simulink model "OFDM_Transreceiver"  (R2020b)
settings: Solver=VariableStepAuto  StartTime=0.0  StopTime=5000  RelTol=1e-3
libraries: xbsIndex_r4 x21, commchan3 x1, commrandsrc3 x1, commsink2 x1
settings Model: Creator=Gokaraan  LastModifiedBy=Gokaraan

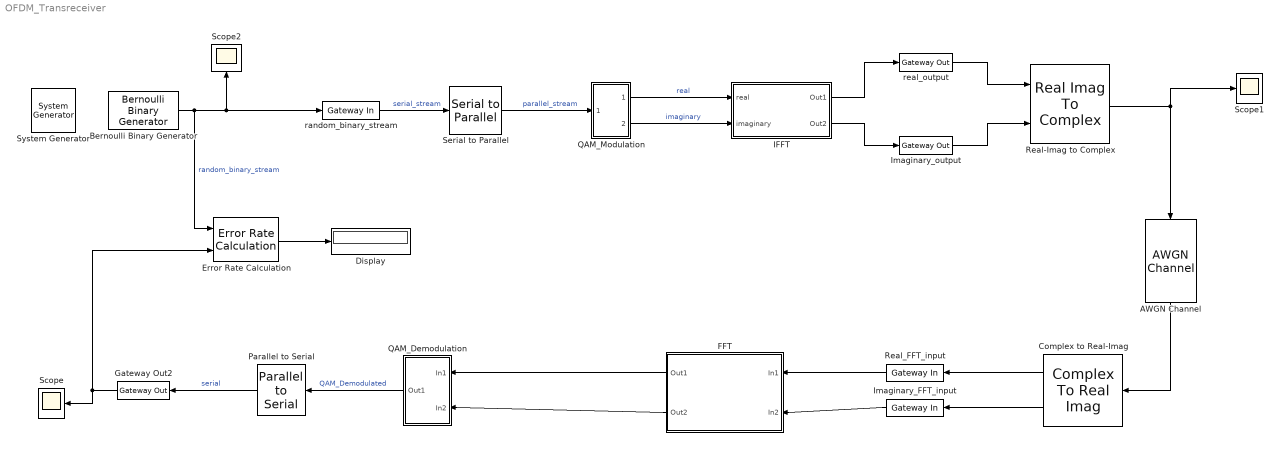
== system OFDM_Transreceiver ==
  " System Generator" : xbsIndex_r4/ System Generator  Tag=genX  xilinxfamily=artix7  part=xc7a35ti  speed=-1L  package=cpg236  synthesis_tool=Vivado  clock_wrapper=Clock Enables  directory=C:/Users/Gokaraan/Documents/Composer/OFDM/HDL  proj_type=Vivado  Synth_file=Vivado Synthesis Defaults  Impl_file=Vivado Implementation Defaults  testbench=off  simulink_period=1  sysclk_period=10  dcm_input_clock_period=10  incr_netlist=off  trim_vbits=Everywhere in SubSystem  dbl_ovrd=According to Block Masks  core_generation=According to Block Masks  run_coregen=off  deprecated_control=off  eval_field=0  block_type=sysgen
  AWGN Channel : commchan3/AWGN Channel  InputProcessing=Columns as channels (frame based)  seed=67  noiseMode="Signal to noise ratio  (SNR)"  EbNodB=10  EsNodB=10  SNRdB=70  bitsPerSym=1  Ps=1  Tsym=1  variance=1
  Bernoulli Binary Generator : commrandsrc3/Bernoulli Binary Generator  ProbabilityOfZero=0.5  SeedSource=Parameter  Seed=61  SampleTime=1  SamplesPerFrame=1  OutputDataType=double  SimulateUsing=Interpreted execution
  Complex to Real-Imag : ComplexToRealImag
  Display : Display
  Error Rate Calculation : commsink2/Error Rate Calculation  N=1672  st_delay=700  cp_mode=Entire frame  subframe=[]  PMode=Port  WsName=ErrorVec  RsMode2=off  stop=off  numErr=100  maxBits=1e6
      settings: SourceProductName=Communications Toolbox
  FFT : Subsystem
  Gateway Out2 : xbsIndex_r4/Gateway Out  inherit_from_input=off  hdl_port=on  rows=1  columns=1  UseAsDAC=off  DACChannel='1'  interface=None  automatic_assignment=on  address_offset=hex2dec('00')  intf_name=''  intf_description=''  timing_constraint=None  locs_specified=off  LOCs={}  io_standard={}  block_type=gatewayout
  IFFT : Subsystem
  Imaginary_FFT_input : xbsIndex_r4/Gateway In  gui_display_data_type=Fixed-point  arith_type="Signed  (2's comp)"  n_bits=16  bin_pt=15  preci_type=Single  exp_width=8  frac_width=24  rows=1  columns=1  quantization="Round  (unbiased: +/- Inf)"  overflow=Saturate  period=4  UseAsADC=off  ADCChannel='1'  interface=None  automatic_assignment=on  address_offset=hex2dec('00')  intf_name=''  intf_description=''  default_value=0  timing_constraint=None  locs_specified=off  LOCs={}  io_standard={}  inherit_from_input=off  hdl_port=on  dbl_ovrd=off  block_type=gatewayin
  Imaginary_output : xbsIndex_r4/Gateway Out  inherit_from_input=off  hdl_port=on  rows=1  columns=1  UseAsDAC=off  DACChannel='1'  interface=None  automatic_assignment=on  address_offset=hex2dec('00')  intf_name=''  intf_description=''  timing_constraint=None  locs_specified=off  LOCs={}  io_standard={}  block_type=gatewayout
  Parallel to Serial : xbsIndex_r4/Parallel to Serial  output_order=Least Significant Word First  arith_type=Unsigned  output_bits=1  bin_pt=0  rst=off  en=off  latency=1  dbl_ovrd=off  block_type=p2s
      settings: infoedit=Each sample presented at the input becomes several samples presented serially at the output.
  QAM_Demodulation : Subsystem
  QAM_Modulation : Subsystem
  Real-Imag to Complex : RealImagToComplex
  Real_FFT_input : xbsIndex_r4/Gateway In  gui_display_data_type=Fixed-point  arith_type="Signed  (2's comp)"  n_bits=16  bin_pt=15  preci_type=Single  exp_width=8  frac_width=24  rows=1  columns=1  quantization="Round  (unbiased: +/- Inf)"  overflow=Saturate  period=4  UseAsADC=off  ADCChannel='1'  interface=None  automatic_assignment=on  address_offset=hex2dec('00')  intf_name=''  intf_description=''  default_value=0  timing_constraint=None  locs_specified=off  LOCs={}  io_standard={}  inherit_from_input=off  hdl_port=on  dbl_ovrd=off  block_type=gatewayin
  Scope : Scope
  Scope1 : Scope
  Scope2 : Scope
  Serial to Parallel : xbsIndex_r4/Serial to Parallel  input_order=Least Significant Word First  arith_type=Unsigned  output_bits=4  bin_pt=0  rst=off  en=off  latency=1  dbl_ovrd=off  block_type=s2p
      settings: infoedit=Groups of samples presented serially at the input become single samples presented at the output.
  random_binary_stream : xbsIndex_r4/Gateway In  gui_display_data_type=Fixed-point  arith_type=Unsigned  n_bits=1  bin_pt=0  preci_type=Single  exp_width=8  frac_width=24  rows=1  columns=1  quantization="Round  (unbiased: +/- Inf)"  overflow=Saturate  period=1  UseAsADC=off  ADCChannel='1'  interface=None  automatic_assignment=on  address_offset=hex2dec('00')  intf_name=''  intf_description=''  default_value=0  timing_constraint=None  locs_specified=off  LOCs={}  io_standard={}  inherit_from_input=off  hdl_port=on  dbl_ovrd=off  block_type=gatewayin
  real_output : xbsIndex_r4/Gateway Out  inherit_from_input=off  hdl_port=on  rows=1  columns=1  UseAsDAC=off  DACChannel='1'  interface=None  automatic_assignment=on  address_offset=hex2dec('00')  intf_name=''  intf_description=''  timing_constraint=None  locs_specified=off  LOCs={}  io_standard={}  block_type=gatewayout
  wires:
  Bernoulli Binary Generator/1 -> Error Rate Calculation/1, random_binary_stream/1, Scope2/1  "random_binary_stream"
  Complex to Real-Imag/2 -> Imaginary_FFT_input/1
  random_binary_stream/1 -> Serial to Parallel/1  "serial_stream"
  Complex to Real-Imag/1 -> Real_FFT_input/1
  Imaginary_output/1 -> Real-Imag to Complex/2
  AWGN Channel/1 -> Complex to Real-Imag/1
  Real-Imag to Complex/1 -> Scope1/1, AWGN Channel/1
  Parallel to Serial/1 -> Gateway Out2/1  "serial"
  Gateway Out2/1 -> Scope/1, Error Rate Calculation/2
  real_output/1 -> Real-Imag to Complex/1
  Error Rate Calculation/1 -> Display/1
  Serial to Parallel/1 -> QAM_Modulation/1(In1)  "parallel_stream"
  QAM_Modulation/1(Out1) -> IFFT/1(real)  "real"
  QAM_Modulation/2(Out2) -> IFFT/2(imaginary)  "imaginary"
  IFFT/1(Out1) -> real_output/1
  IFFT/2(Out2) -> Imaginary_output/1
  Real_FFT_input/1 -> FFT/1(In1)
  Imaginary_FFT_input/1 -> FFT/2(In2)
  FFT/1(Out1) -> QAM_Demodulation/1(In1)
  FFT/2(Out2) -> QAM_Demodulation/2(In2)
  QAM_Demodulation/1(Out1) -> Parallel to Serial/1  "QAM_Demodulated"

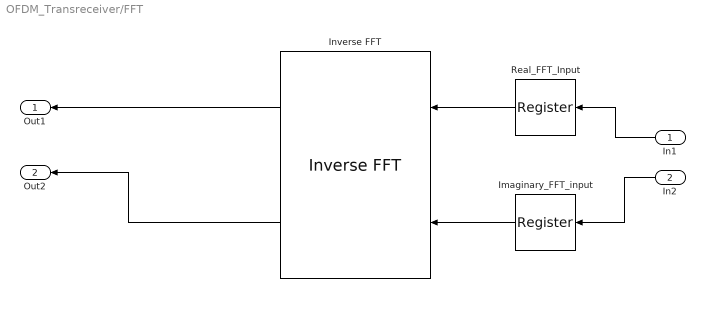
== system OFDM_Transreceiver/FFT ==
  In1 : Inport
  In2 : Inport  Port=2
  Imaginary_FFT_input : xbsIndex_r4/Register  init=0  rst=off  en=off  dbl_ovrd=off  block_type=register
  Inverse FFT : xbsIndex_r4/Inverse FFT  infoeditControl=Hardware notes: This block implements a burst IO radix-2 architecture if the <b><i>Optimize for</i></b> parameter is selected as <b><i>Resources</i></b>, and the input sample period is 8 times slower than the system sample period; otherwise a pipeline streaming architecture will be used.  transform_length=64  scale_result_by_fft_length=off  bit_reversed_order=off  optimizegoal=Performance  start_frame=off  simulation_type=fast_sim  simulation_model=sysgen:InverseFFT_Macro  latency=1  block_type=xfft_inverse
  Real_FFT_Input : xbsIndex_r4/Register  init=0  rst=off  en=off  dbl_ovrd=off  block_type=register
  Out1 : Outport
  Out2 : Outport  Port=2
  wires:
  Imaginary_FFT_input/1 -> Inverse FFT/2
  Real_FFT_Input/1 -> Inverse FFT/1
  In1/1 -> Real_FFT_Input/1
  Inverse FFT/1 -> Out1/1
  Inverse FFT/2 -> Out2/1
  In2/1 -> Imaginary_FFT_input/1

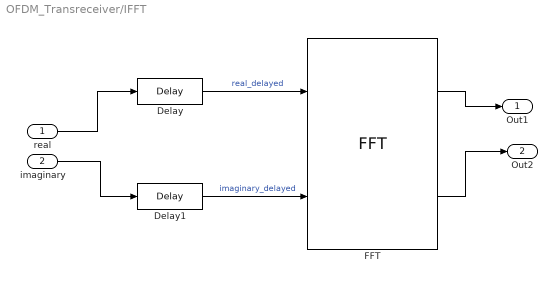
== system OFDM_Transreceiver/IFFT ==
  real : Inport
  imaginary : Inport  Port=2
  Delay : xbsIndex_r4/Delay  rst=off  infoeditControl=Selection of Reset will increase slice count due to use of real FFs and instead of SRLs  en=off  latency=1  reg_retiming=off  dbl_ovrd=off  block_type=delay
  Delay1 : xbsIndex_r4/Delay  rst=off  infoeditControl=Selection of Reset will increase slice count due to use of real FFs and instead of SRLs  en=off  latency=1  reg_retiming=off  dbl_ovrd=off  block_type=delay
  FFT : xbsIndex_r4/FFT  infoeditControl=Hardware notes: This block implements a burst IO radix-2 architecture if the <b><i>Optimize for</i></b> parameter is selected as <b><i>Resources</i></b>, and the input sample period is 8 times slower than the system sample period; otherwise a pipeline streaming architecture will be used.  transform_length=64  scale_result_by_fft_length=off  bit_reversed_order=off  optimizegoal=Performance  start_frame=off  simulation_type=fast_sim  simulation_model=sysgen:ForwardFFT_Macro  latency=1  block_type=xfft_forward
  Out1 : Outport
  Out2 : Outport  Port=2
  wires:
  Delay1/1 -> FFT/2  "imaginary_delayed"
  Delay/1 -> FFT/1  "real_delayed"
  imaginary/1 -> Delay1/1
  FFT/2 -> Out2/1
  real/1 -> Delay/1
  FFT/1 -> Out1/1

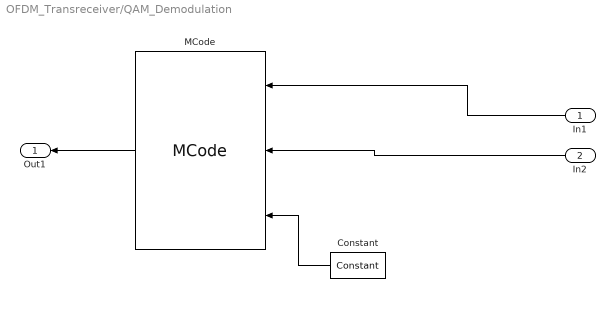
== system OFDM_Transreceiver/QAM_Demodulation ==
  In1 : Inport
  In2 : Inport  Port=2
  Constant : xbsIndex_r4/Constant  const=0.25  gui_display_data_type=Fixed-point  arith_type=Signed (2's comp)  n_bits=5  bin_pt=3  preci_type=Single  exp_width=8  frac_width=24  explicit_period=off  period=1  equ=P=C  opselect=C  inp2=PCIN>>17  opr=+  inp1=P  carry=CIN  dbl_ovrd=off  block_type=constant
  MCode : xbsIndex_r4/MCode  mfname=QAM16_DEM  explicit_period=off  period=1  inputsTable={'boundInpExpr'=>['','',''],'inputs'=>['I','Q','Thrd']}  outputsTable={'outputs'=>['B'],'suppressOut'=>['off']}  enable_stdout=off  enable_debug=off  suppress_output=on  defparams={}  hide_port_list={}  dbl_ovrd=off  block_type=mcode
  Out1 : Outport
  wires:
  Constant/1 -> MCode/3
  In1/1 -> MCode/1
  MCode/1 -> Out1/1
  In2/1 -> MCode/2

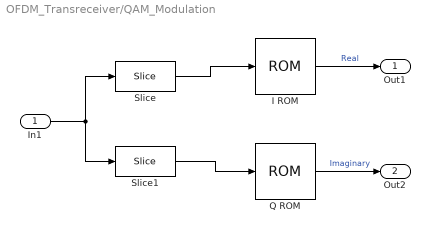
== system OFDM_Transreceiver/QAM_Modulation ==
  In1 : Inport
  I ROM : xbsIndex_r4/ROM  depth=4  initVector=[-3 +3 -1 +1]/3  distributed_mem=Block RAM  rst=off  init_reg=0  en=off  latency=1  gui_display_data_type=Fixed-point  arith_type="Signed  (2's comp)"  n_bits=16  bin_pt=15  preci_type=Single  exp_width=8  frac_width=24  optimize=Area  use_rpm=on  dbl_ovrd=off  simulation_type=fast_sim  block_type=sprom
  Q ROM : xbsIndex_r4/ROM  depth=4  initVector=[-3 +3 -1 +1]/3  distributed_mem=Block RAM  rst=off  init_reg=0  en=off  latency=1  gui_display_data_type=Fixed-point  arith_type="Signed  (2's comp)"  n_bits=16  bin_pt=15  preci_type=Single  exp_width=8  frac_width=24  optimize=Area  use_rpm=on  dbl_ovrd=off  simulation_type=fast_sim  block_type=sprom
  Slice : xbsIndex_r4/Slice  nbits=2  boolean_output=off  mode=Lower Bit Location + Width  bit1=0  base1=MSB of Input  bit0=0  base0=LSB of Input  dbl_ovrd=off  block_type=slice
  Slice1 : xbsIndex_r4/Slice  nbits=2  boolean_output=off  mode=Upper Bit Location + Width  bit1=0  base1=MSB of Input  bit0=0  base0=LSB of Input  dbl_ovrd=off  block_type=slice
  Out1 : Outport
  Out2 : Outport  Port=2
  wires:
  In1/1 -> Slice1/1, Slice/1
  Slice1/1 -> Q ROM/1
  I ROM/1 -> Out1/1  "Real"
  Slice/1 -> I ROM/1
  Q ROM/1 -> Out2/1  "Imaginary"
